simulink model "IFSSIM_TireSuspension"  (R2025b)
settings: Solver=ode1  StartTime=0  StopTime=inf  FixedStep=0.0010416666666666671  RelTol=1e-3
undefined symbols (not defined in the file or in its folder): IFSSIM_aF, IFSSIM_arbF, IFSSIM_arbR, IFSSIM_bR, IFSSIM_camF, IFSSIM_camR, IFSSIM_cgainF, IFSSIM_cgainR, IFSSIM_CoGH, IFSSIM_Crr, IFSSIM_cw, IFSSIM_FzF, IFSSIM_FzR, IFSSIM_Iw, IFSSIM_kwF, IFSSIM_kwR, IFSSIM_L0, IFSSIM_mu, IFSSIM_Ppres, IFSSIM_Rw, IFSSIM_tF, IFSSIM_tR, IFSSIM_Ts, IFSSIM_vreg, IFSSIM_wreg
libraries: vehdynlibtire x1
settings Model: Creator=raulmoran  LastModifiedBy=raulmoran
settings DataIOCC: SignalLoggingName=tsLog

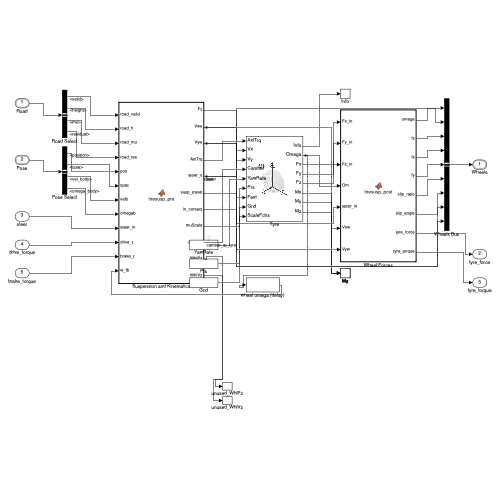
[thumbnail: Simulink's stored preview of the top-level diagram]
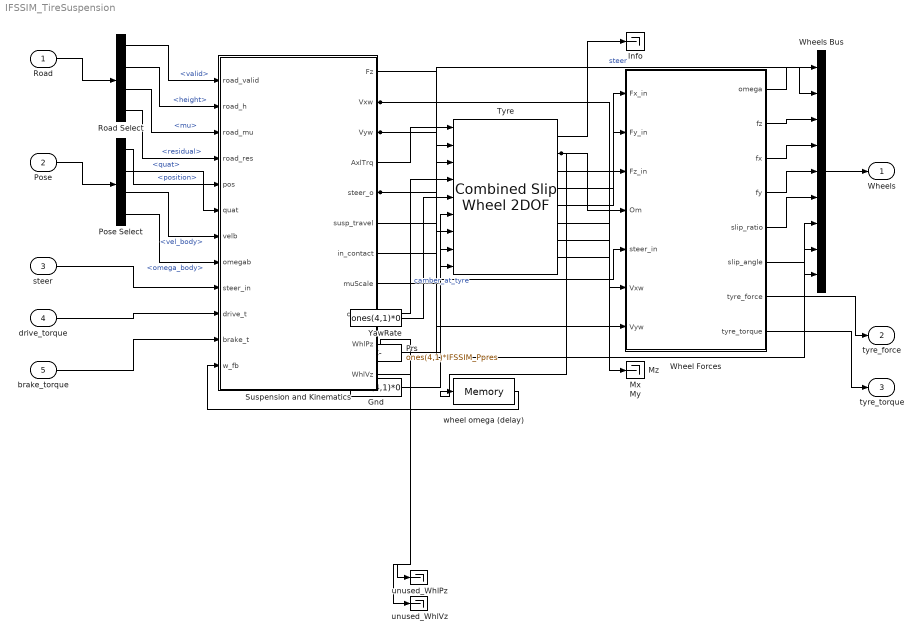
== system IFSSIM_TireSuspension ==
  Road : Inport  OutDataTypeStr=Bus: IFSSIM_RoadBus  BusOutputAsStruct=on
  Pose : Inport  Port=2  OutDataTypeStr=Bus: IFSSIM_PoseBus  BusOutputAsStruct=on
  steer : Inport  Port=3  PortDimensions=4
  drive_torque : Inport  Port=4  PortDimensions=4
  brake_torque : Inport  Port=5  PortDimensions=4
  Gnd : Constant  Value=ones(4,1)*0
  Info : Terminator
  Mx : Terminator
  My : Terminator
  Mz : Terminator
  Pose Select : BusSelector  OutputSignals=position,quat,vel_body,omega_body
  Prs : Constant  Value=ones(4,1)*IFSSIM_Ppres
  Road Select : BusSelector  OutputSignals=valid,height,mu,residual
  Suspension and Kinematics : MATLAB Function  TreatAsAtomicUnit=on
  Tyre : vehdynlibtire/Combined Slip Wheel 2DOF  tireType=External file  tireParamSet=ifssim_tyre.mat  vertType=None  plySteer=off  turnslip=off  BrakeType=None  mu_static=.3  mu_kinetic=.2  drum_abore=0.0508  drum_a=0.123  drum_c=0.212  drum_r=0.15  drum_theta1=0  drum_theta2=126  disk_abore=.05  Rm=.177  num_pads=2  brake_p_bpt=[1 11.4736842105263 21.9473684210526 32.4210526315789 42.8947368421053 53.3684210526316 63.8421052631579 74.3157894736842 84.7894736842105 95.2631578947368 105.736842105263 116.210526315789 126.684210526316 137.157894736842 147.631578947368 158.105263157895 168.578947368421 179.052631578947 189.526315789474 200]  brake_n_bpt=[0 52.6315789473684 105.263157894737 157.894736842105 210.526315789474 263.157894736842 315.789473684211 368.421052631579 421.052631578947 473.684210526316 526.315789473684 578.947368421053 631.578947368421 684.210526315789 736.842105263158 789.473684210526 842.105263157895 894.736842105263 947.368421052632 1000]  f_brake_t=[43.4900602404453 42.5056030554862 41.5350898940194 40.5780454442085 39.6340111501808 38.7025443887544 37.7832176914519 36.8756180088306 35.9793460143796 35.0940154454303 34.2192524787115 33.3546951383474 32.4999927342521 31.6548053290159 30.8188032315107 29.991666515561 29.1730845621415 28.362755623661 27.5603864089927 26.765691687993;498.991217495636 487.695866636631 476.560505099801 465.579679307235 454.748127933653 444.060772460445 433.51270824929 423.099196101319 412.81565427025 402.657650900201 392.620896861006 382.701238955775 372.894653477208 363.197240090814 353.605216024701 344.114910546964 334.722759712992 325.425301366216 316.219170376863 307.10109410434;954.492374750826 932.886130217776 911.585920305583 890.581313170261 869.862244717126 849.419000532136 829.242198807128 809.322774193808 789.651962526121 770.221286354971 751.0225412433 732.047782773203 713.289314220164 694.739674852612 676.391628817892 658.238154578366 640.272434863842 622.48784710877 604.877954344734 587.436496520688;1409.99353200602 1378.07639379892 1346.61133551136 1315.58294703329 1284.9763615006 1254.77722860383 1224.97168936497 1195.5463522863 1166.48827078199 1137.78492180974 1109.42418562559 1081.39432659063 1053.68397496312 1026.28210961441 999.178041611083 972.361398609768 945.822110014692 919.550392851325 893.536738312604 867.771898937035;1865.49468926121 1823.26665738007 1781.63675071715 1740.58458089631 1700.09047828407 1660.13545667552 1620.7011799228 1581.76993037878 1543.32457903786 1505.34855726451 1467.82583000789 1430.74087040806 1394.07863570608 1357.82454437621 1321.96445440427 1286.48464264117 1251.37178516554 1216.61293859388 1182.19552228048 1148.10730135338;2320.9958465164 2268.45692096121 2216.66216592293 2165.58621475934 2115.20459506754 2065.49368474721 2016.43067048064 1967.99350847127 1920.16088729373 1872.91219271928 1826.22747439018 1780.08741422549 1734.47329644903 1689.36697913801 1644.75086719747 1600.60788667257 1556.92146031639 1513.67548433643 1470.85430624835 1428.44270376973;2776.49700377159 2713.64718454235 2651.68758112871 2590.58784862237 2530.31871185102 2470.8519128189 2412.16016103848 2354.21708656376 2296.9971955496 2240.47582817405 2184.62911877248 2129.43395804292 2074.86795719199 2020.9094138998 1967.53727999066 1914.73113070398 1862.47113546724 1810.73803007899 1759.51309021622 1708.77810618608;3231.99816102678 3158.8374481235 3086.71299633449 3015.58948248539 2945.43282863449 2876.21014089059 2807.88965159632 2740.44066465625 2673.83350380547 2608.03946362882 2543.03076315477 2478.78050186034 2415.26261793494 2352.4518486616 2290.32369278385 2228.85437473538 2168.02081061809 2107.80057582154 2048.17187418409 1989.11350860242;3687.49931828197 3604.02771170464 3521.73841154027 3440.59111634842 3360.54694541796 3281.56836896228 3203.61914215416 3126.66424274874 3050.66981206134 2975.60309908359 2901.43240753707 2828.12704567777 2755.6572786779 2683.9942834234 2613.11010557704 2542.97761876678 2473.57048576894 2404.8631215641 2336.83065815196 2269.44891101877;4143.00047553716 4049.21797528579 3956.76382674606 3865.59275021144 3775.66106220143 3686.92659703397 3599.34863271199 3512.88782084123 3427.50612031721 3343.16673453836 3259.83405191936 3177.4735894952 3096.05193942085 3015.5367181852 2935.89651837023 2857.10086279818 2779.12016091979 2701.92566730665 2625.48944211983 2549.78431343512;4598.50163279235 4494.40823886693 4391.78924195184 4290.59438407447 4190.77517898491 4092.28482510566 3995.07812326983 3899.11139893372 3804.34242857308 3710.73036999313 3618.23569630166 3526.82013331263 3436.44660016381 3347.079152947 3258.68293116342 3171.22410682959 3084.66983607064 2998.98821304921 2914.1482260877 2830.11971585147;5054.00279004754 4939.59850244808 4826.81465715762 4715.59601793749 4605.88929576838 4497.64305317735 4390.80761382767 4285.3349770262 4181.17873682896 4078.2940054479 3976.63734068395 3876.16667713006 3776.84126090677 3678.62158770879 3581.46934395661 3485.34735086099 ...(+2764 chars)]  NOMPRES=83000  PRESMAX=166000  PRESMIN=41500  FNOMIN=674.4375  FZMAX=6744.375  FZMIN=0  VXLOW=1  KPUMAX=1.5  KPUMIN=-1.5  ALPMAX=1.570796326794897  ALPMIN=-1.570796326794897  CAMMAX=0.2  CAMMIN=-0.2  LONGVL=1000  FxRelFreqLwrLim=200*pi  FyRelFreqLwrLim=200*pi  MyRelFreqLwrLim=100*pi  omegao=0  UNLOADED_RADIUS=IFSSIM_Rw  WIDTH=0.19  RIM_RADIUS=0.12524  ASPECT_RATIO=0.45  MASS=5  IYY=IFSSIM_Iw  br=0  GRAVITY=-9.81  zo=0  zdoto=0  BREFF=0  DREFF=0  FREFF=0  Q_RE0=1  Q_V1=0  Q_V2=0  Q_FZ1=0  Q_FZ2=0  Q_FZ3=0  Q_FCX=0  Q_FCY=0  Q_FCY2=0  PFZ1=0  VERTICAL_STIFFNESS=1000000000  VERTICAL_DAMPING=0  BOTTOM_OFFST=0  BOTTOM_STIFF=0  Q_CAM1=0  Q_CAM2=0  Q_CAM3=0  Q_FYS1=0  Q_FYS2=0  Q_FYS3=0  LONGITUDINAL_STIFFNESS=96312.41321625  LATERAL_STIFFNESS=44063.25  PCFX1=0  PCFX2=0  PCFX3=0  PCFY1=0  PCFY2=0  PCFY3=0  Q_RA1=0  Q_RA2=0  Q_RB1=0  Q_RB2=0  PCX1=1.46  PDX1=1.4  PDX2=-0.15  PDX3=0  PEX1=-0.5  PEX2=0  PEX3=0  PEX4=0  PKX1=28.560812  PKX2=0  PKX3=0  PHX1=0  PHX2=0  PVX1=0  PVX2=0  PPX1=0  PPX2=0  PPX3=0  PPX4=0  RBX1=9.171685466801819  RBX2=0  RBX3=0  RCX1=1  REX1=0  REX2=0  RHX1=0  QSX1=0  QSX2=0  QSX3=0  QSX4=0  QSX5=0  QSX6=0  QSX7=0  QSX8=0  QSX9=0  QSX10=0  QSX11=0  QSX12=0  QSX13=0  QSX14=0  PPMX1=0  PCY1=1.4  PDY1=1.4  PDY2=-0.15  PDY3=0  PEY1=-0.3  PEY2=0  PEY3=0  PEY4=0  PEY5=0  PKY1=-24.5  PKY2=2  PKY3=0  PKY4=2  PKY5=0  PKY6=0  PKY7=0  PHY1=0  PHY2=0  PVY1=0  PVY2=0  PVY3=0  PVY4=0  PPY1=0  PPY2=0  PPY3=0  PPY4=0  PPY5=0  RBY1=10.84762403199215  RBY2=0  RBY3=0  RBY4=0  RCY1=1  REY1=0  REY2=0  RHY1=0  RHY2=0  RVY1=0  RVY2=0  RVY3=0  RVY4=0  RVY5=0  RVY6=0  QSY1=0  QSY2=0  QSY3=0  QSY4=0  QSY5=0  QSY6=0  QSY7=0  QSY8=0  QBZ1=0  QBZ2=0  QBZ3=0  QBZ4=0  QBZ5=0  QBZ6=0  QBZ9=0  QBZ10=0  QCZ1=0  QDZ1=0  QDZ2=0  QDZ3=0  QDZ4=0  QDZ6=0  QDZ7=0  QDZ8=0  QDZ9=0  QDZ10=0  QDZ11=0  QEZ1=0  QEZ2=0  QEZ3=0  QEZ4=0  QEZ5=0  QHZ1=0  QHZ2=0  QHZ3=0  QHZ4=0  PPZ1=0  PPZ2=0  SSZ1=0  SSZ2=0  SSZ3=0  SSZ4=0  PDXP1=0  PDXP2=0  PDXP3=0  PKYP1=0  PDYP1=0  PDYP2=0  PDYP3=0  PDYP4=0  PHYP1=0  PHYP2=0  PHYP3=0  PHYP4=0  PECP1=0  PECP2=0  QDTP1=0  QCRP1=0  QCRP2=0  QBRP1=0  QDRP1=0  QDRP2=0  aMode=2
  Wheel Forces : MATLAB Function  TreatAsAtomicUnit=on
  Wheels Bus : BusCreator  Inputs=9  OutDataTypeStr=Bus: IFSSIM_WheelsBus  NonVirtualBus=on
  YawRate : Constant  Value=ones(4,1)*0
  unused_WhlPz : Terminator
  unused_WhlVz : Terminator
  wheel omega (delay) : Memory
  Wheels : Outport  OutDataTypeStr=Bus: IFSSIM_WheelsBus
  tyre_force : Outport  Port=2  PortDimensions=3
  tyre_torque : Outport  Port=3  PortDimensions=3
  wires:
  Road/1 -> Road Select/1
  Pose/1 -> Pose Select/1
  Wheels Bus/1 -> Wheels/1
  Road Select/1 -> Suspension and Kinematics/1(road_valid)  "<valid>"
  Road Select/2 -> Suspension and Kinematics/2(road_h)  "<height>"
  Road Select/3 -> Suspension and Kinematics/3(road_mu)  "<mu>"
  Road Select/4 -> Suspension and Kinematics/4(road_res)  "<residual>"
  Pose Select/1 -> Suspension and Kinematics/5(pos)  "<position>"
  Pose Select/2 -> Suspension and Kinematics/6(quat)  "<quat>"
  Pose Select/3 -> Suspension and Kinematics/7(velb)  "<vel_body>"
  Pose Select/4 -> Suspension and Kinematics/8(omegab)  "<omega_body>"
  steer/1 -> Suspension and Kinematics/9(steer_in)
  drive_torque/1 -> Suspension and Kinematics/10(drive_t)
  brake_torque/1 -> Suspension and Kinematics/11(brake_t)
  wheel omega (delay)/1 -> Suspension and Kinematics/12(w_fb)
  Suspension and Kinematics/4(AxlTrq) -> Tyre/1
  Suspension and Kinematics/2(Vxw) -> Tyre/2, Wheel Forces/6(Vxw)
  Suspension and Kinematics/3(Vyw) -> Tyre/3, Wheel Forces/7(Vyw)
  Suspension and Kinematics/9(camber) -> Tyre/4  "camber_at_tyre"
  Suspension and Kinematics/10(WhlPz) -> unused_WhlPz/1
  Suspension and Kinematics/11(WhlVz) -> unused_WhlVz/1
  YawRate/1 -> Tyre/5
  Prs/1 -> Tyre/6
  Suspension and Kinematics/1(Fz) -> Tyre/7
  Gnd/1 -> Tyre/8
  Suspension and Kinematics/8(muScale) -> Tyre/9
  Tyre/1 -> Info/1
  Tyre/2 -> wheel omega (delay)/1, Wheel Forces/4(Om)
  Tyre/3 -> Wheel Forces/1(Fx_in)
  Tyre/4 -> Wheel Forces/2(Fy_in)
  Tyre/5 -> Wheel Forces/3(Fz_in)
  Suspension and Kinematics/5(steer_o) -> Wheel Forces/5(steer_in), Wheels Bus/2  "steer"
  Wheel Forces/1(omega) -> Wheels Bus/1
  Wheel Forces/2(fz) -> Wheels Bus/3
  Wheel Forces/3(fx) -> Wheels Bus/4
  Wheel Forces/4(fy) -> Wheels Bus/5
  Wheel Forces/5(slip_ratio) -> Wheels Bus/6
  Wheel Forces/6(slip_angle) -> Wheels Bus/7
  Suspension and Kinematics/6(susp_travel) -> Wheels Bus/8
  Suspension and Kinematics/7(in_contact) -> Wheels Bus/9
  Wheel Forces/7(tyre_force) -> tyre_force/1
  Wheel Forces/8(tyre_torque) -> tyre_torque/1
  Tyre/6 -> Mx/1
  Tyre/7 -> My/1
  Tyre/8 -> Mz/1

== matlab function IFSSIM_TireSuspension/Wheel Forces ==
  data: Fx_in input size=4; omega output size=4; Fy_in input size=4; Fz_in input size=4; Om input size=4; steer_in input size=4; Vxw input size=4; Vyw input size=4; fz output size=4; fx output size=4; fy output size=4; slip_ratio output size=4; slip_angle output size=4; tyre_force output size=3; tyre_torque output size=3; IFSSIM_aF parameter size=1; IFSSIM_bR parameter size=1; IFSSIM_tF parameter size=1; IFSSIM_tR parameter size=1; IFSSIM_Rw parameter size=1; IFSSIM_vreg parameter size=1; IFSSIM_CoGH parameter size=1
function [omega, fz, fx, fy, slip_ratio, slip_angle, tyre_force, tyre_torque] = ...
         tiresusp_post(Fx_in, Fy_in, Fz_in, Om, steer_in, Vxw, Vyw, IFSSIM_aF, IFSSIM_bR, IFSSIM_tF, IFSSIM_tR, IFSSIM_Rw, IFSSIM_vreg, IFSSIM_CoGH)
%#codegen
% Four wheel forces, in their own wheel frames, assembled into one body-frame
% wrench -- plus the reported per-wheel state.

rx = [ IFSSIM_aF;  IFSSIM_aF; -IFSSIM_bR; -IFSSIM_bR];
ry = [ IFSSIM_tF/2; -IFSSIM_tF/2;  IFSSIM_tR/2; -IFSSIM_tR/2];
Rw = IFSSIM_Rw;

omega = reshape(Om,    4, 1);
fx    = reshape(Fx_in, 4, 1);
fy    = reshape(Fy_in, 4, 1);
fz    = reshape(Fz_in, 4, 1);

slip_ratio = zeros(4,1);  slip_angle = zeros(4,1);
F_sum = zeros(3,1);       M_sum      = zeros(3,1);

for i = 1:4
    % Slip is REPORTED here, not used. The tyre block computes its own
    % internally, with relaxation; this is the algebraic value, recomputed
    % for telemetry so the bus still carries the quantity it always did.
    vref = max(abs(Vxw(i)), IFSSIM_vreg);
    slip_ratio(i) = (omega(i)*Rw - Vxw(i)) / vref;
    slip_angle(i) = atan2(Vyw(i), vref);

    % Wheel frame -> body frame. Fx acts along the wheel, Fy across it, and
    % the wheel is rotated by the steer angle relative to the body.
    d  = steer_in(i);
    cd = cos(d); sd = sin(d);
    Fb = [fx(i)*cd - fy(i)*sd; fx(i)*sd + fy(i)*cd; fz(i)];
    F_sum = F_sum + Fb;

    % The tyre force acts at the CONTACT PATCH, on the road, not at the CoG.
    % That arm IS load transfer: it is what turns a lateral force into a roll
    % moment and a longitudinal force into a pitch moment.
    %
    % This used to be [rx; ry; 0], and the reason it survived so long is that
    % a zero z still gives the RIGHT answer for three of the six terms. Yaw
    % (rx*fy - ry*fx) has no z in it at all, and the roll and pitch from the
    % VERTICAL loads (ry*fz, -rx*fz) do not either. So the car rolled
    % correctly whenever something else rolled it -- which is every test that
    % imposes a body rate. What it could not do was roll ITSELF: the two
    % missing terms, -rz*fy and +rz*fx, are precisely the ones by which the
    % tyres act on the body. Measured before the fix: 0.000000 rad of roll in
    % a 1.2 g corner, and load transfer at 0.1% of what m*a*h/t requires.
    %
    % Taking the arm all the way to the ground puts the roll centre at ground
    % level, so every newton of lateral transfer goes through the springs and
    % none through the suspension links. That is a real assumption and it is
    % stated here rather than hidden: this model HAS no links -- no wishbones,
    % no instantaneous centres -- so a non-zero roll centre would not be a
    % better number, it would be an invented one. It costs less than it
    % sounds: the TOTAL transfer is m*a*h/t whatever the roll centre does.
    % What a real one would change is the elastic/geometric split, and with
    % it the roll ANGLE and the transient, not the steady-state load split.
    %
    % The height is held constant at the static CoG height. Tracking ride
    % height through suspension travel would be a centimetre of correction on
    % a 34 cm arm, sitting on top of a CoG height nobody has measured.
    M_sum = M_sum + cross([rx(i); ry(i); -IFSSIM_CoGH], Fb);
end

tyre_force  = F_sum;
tyre_torque = M_sum;
end

== matlab function IFSSIM_TireSuspension/Suspension and Kinematics ==
  data: road_valid input size=4; Fz output size=4; road_h input size=4; road_mu input size=4; road_res input size=4; pos input size=3; quat input size=4; velb input size=3; omegab input size=3; steer_in input size=4; drive_t input size=4; brake_t input size=4; w_fb input size=4; Vxw output size=4; Vyw output size=4; AxlTrq output size=4; steer_o output size=4; susp_travel output size=4; in_contact output size=4; muScale output size=[27 4]; camber output size=4; WhlPz output size=4; WhlVz output size=4; IFSSIM_arbF parameter size=1; IFSSIM_arbR parameter size=1; IFSSIM_Ts parameter size=1; IFSSIM_Iw parameter size=1; IFSSIM_wreg parameter size=1; IFSSIM_aF parameter size=1; IFSSIM_bR parameter size=1; IFSSIM_tF parameter size=1; IFSSIM_tR parameter size=1; IFSSIM_Rw parameter size=1; IFSSIM_kwF parameter size=1; IFSSIM_kwR parameter size=1; IFSSIM_cw parameter size=1; IFSSIM_L0 parameter size=1; IFSSIM_FzF parameter size=1; IFSSIM_FzR parameter size=1; IFSSIM_camF parameter size=1; IFSSIM_camR parameter size=1; IFSSIM_cgainF parameter size=1; IFSSIM_cgainR parameter size=1; IFSSIM_mu parameter size=1; IFSSIM_Crr parameter size=1
function [Fz, Vxw, Vyw, AxlTrq, steer_o, susp_travel, in_contact, muScale, camber, WhlPz, WhlVz] = ...
         tiresusp_pre(road_valid, road_h, road_mu, road_res, pos, quat, velb, omegab, steer_in, drive_t, brake_t, w_fb, IFSSIM_arbF, IFSSIM_arbR, IFSSIM_Ts, IFSSIM_Iw, IFSSIM_wreg, IFSSIM_aF, IFSSIM_bR, IFSSIM_tF, IFSSIM_tR, IFSSIM_Rw, IFSSIM_kwF, IFSSIM_kwR, IFSSIM_cw, IFSSIM_L0, IFSSIM_FzF, IFSSIM_FzR, IFSSIM_camF, IFSSIM_camR, IFSSIM_cgainF, IFSSIM_cgainR, IFSSIM_mu, IFSSIM_Crr)
%#codegen
% Suspension load and contact-patch kinematics for four corners, plus the
% axle torque that drives the tyre block.
%
% Wheel order FL, FR, RL, RR. Body frame ISO 8855: x forward, y LEFT, z up.

Rw = IFSSIM_Rw;

% Wheel positions in the body frame, at CoG height. y is POSITIVE LEFT, so the
% left wheels take +track/2. Getting this backwards mirrors the car and is
% almost impossible to see in a lap time.
rx = [ IFSSIM_aF;  IFSSIM_aF; -IFSSIM_bR; -IFSSIM_bR];
ry = [ IFSSIM_tF/2; -IFSSIM_tF/2;  IFSSIM_tR/2; -IFSSIM_tR/2];
Fz_static = [IFSSIM_FzF; IFSSIM_FzF; IFSSIM_FzR; IFSSIM_FzR];

q = quat / max(norm(quat), eps);
R = q2r(q);                      % body -> world
vel_world   = R * velb;
omega_world = R * omegab;

Fz      = zeros(4,1);  Vxw     = zeros(4,1);  Vyw        = zeros(4,1);
AxlTrq  = zeros(4,1);  steer_o = zeros(4,1);  susp_travel= zeros(4,1);
camber  = zeros(4,1);
% What the VDB suspension block wants, if it is in the model: displacement
% from the static ride position in a z-DOWN frame, so positive is droop and
% our compression-positive delta is its negative. Measured, see
% docs/vdb_step1_port_semantics.md -- feeding it a ride height instead of a
% displacement is what made the first attempt return 2568 N a wheel.
WhlPz   = zeros(4,1);  WhlVz = zeros(4,1);
in_contact = zeros(4,1);  muScale = ones(27,4);

% ---- suspension deflection, all four corners at once ----------------
% This has to be a separate pass. An anti-roll bar reacts the DIFFERENCE in
% deflection across an axle, so no corner's vertical load can be known until
% both corners of its axle are.
delta  = zeros(4,1);
ddelta = zeros(4,1);
for i = 1:4
    r_w = R * [rx(i); ry(i); 0];
    p_w = pos + r_w;                      % corner position, world
    % delta > 0 means compressed relative to static ride height.
    gap       = p_w(3) - (road_h(i) + Rw);    % attachment above wheel centre
    delta(i)  = IFSSIM_L0 - gap;
    % Compression RATE is the downward velocity of this corner. Using the
    % corner velocity rather than the CoG velocity is what makes roll and
    % pitch damping appear at all.
    v_corner  = vel_world + cross(omega_world, r_w);
    ddelta(i) = -v_corner(3);
end

% ---- anti-roll bars -------------------------------------------------
% A bar carries K_arb times the roll angle of its axle, delivered as a force
% couple across the track: dF = K_arb*(dL - dR)/t^2, up on the compressed
% side and down on the other, summing to zero so it adds no heave stiffness.
%
% These are not a detail. They are the ONLY thing that makes the front and
% rear roll stiffnesses differ, and that difference is the car's balance.
% With four equal springs and equal tracks -- which is what this model had --
% lateral load transfer splits exactly 50.0/50.0 at every steer angle and
% nothing can move it, so the car can be neither understeering nor
% oversteering by construction. See ifssim_params for how the bar rates come
% out of RollStiffnessFront/Rear, which until now were read by nothing.
arbF = IFSSIM_arbF * (delta(1) - delta(2)) / (IFSSIM_tF*IFSSIM_tF);
arbR = IFSSIM_arbR * (delta(3) - delta(4)) / (IFSSIM_tR*IFSSIM_tR);
arb  = [arbF; -arbF; arbR; -arbR];

% ---- camber -----------------------------------------------------------
% Inclination each tyre sees: its static setting, plus the share of body roll
% the geometry does NOT take back out. Camber gain 1.0 keeps the wheel
% upright through the corner; a real double wishbone falls short of that.
%
% Roll comes from the quaternion the chassis already integrates, so this is
% the roll the car ACTUALLY has -- not the algebraic estimate the design
% model has to make. That is the one place the plant is now ahead of it.
%
% It is wired to the tyre block's Camber input, which this model used to hold
% at a constant zero. The tyre does not yet RESPOND to it: the camber
% coefficients in the Magic Formula set are zeroed, because nobody has put
% this tyre on a rig and inventing PDY3 would be inventing grip. The
% kinematics are real and arrive at the tyre; the tyre's answer to them is
% the part still waiting on data.
%
% The two terms mirror DIFFERENTLY, and getting that backwards is the easy
% mistake. In the ISO tyre axis system y points left on BOTH wheels, so:
%
%   static camber is symmetric in space -- the tops lean toward each other --
%   and therefore reads with OPPOSITE sign on the two sides (sgnOut);
%
%   roll tilts both wheels the SAME way in space, so it reads with the SAME
%   sign on both, and must stay OUTSIDE the mirror.
%
% This used to apply the static setting uniformly to all four and mirror the
% roll term -- exactly inverted, on both counts. It changed no force, because
% the camber coefficients are zeroed, and it would have changed every one of
% them the day rig data arrives. The structure here is not argued from the
% convention: it is what the VDB double-wishbone block measurably does
% (see vdb_camber_mask), and the two now agree to 3e-10 deg.
%
% The OVERALL SIGN of gamma is still unpinned. Nothing in this plant can
% settle it while the Magic Formula camber terms are zero -- there is no
% observable to check it against. It wants fixing against rig data, not
% against an argument.
rollAng = atan2(2*(q(1)*q(2) + q(3)*q(4)), 1 - 2*(q(2)*q(2) + q(3)*q(3)));
sgnOut  = [-1; 1; -1; 1];
camber  = sgnOut .* [IFSSIM_camF; IFSSIM_camF; IFSSIM_camR; IFSSIM_camR] + ...
          (1 - [IFSSIM_cgainF; IFSSIM_cgainF; IFSSIM_cgainR; IFSSIM_cgainR]) * rollAng;

for i = 1:4
    r_b = [rx(i); ry(i); 0];
    r_w = R * r_b;
    p_w = pos + r_w;                      % corner position, world

    kw_i = IFSSIM_kwF; if i > 2, kw_i = IFSSIM_kwR; end
    Fz_i = Fz_static(i) + kw_i * delta(i) + IFSSIM_cw * ddelta(i) + arb(i);

    % A tyre cannot pull the road. Clamping here is what lets a wheel lift
    % in a corner instead of generating negative grip.
    if Fz_i < 0, Fz_i = 0; end
    % Contact needs the platform to have actually CHARACTERISED the ground,
    % not merely to have hit something with one ray.
    %
    % A NEGATIVE residual is the platform saying it could not fit a plane at
    % all - fewer than three of its rays hit - so it does not know what is
    % under this wheel. Standing on an answer nobody has is how a wheel ends
    % up loaded against geometry that is not there.
    %
    % A LARGE residual is a different thing entirely and deliberately does NOT
    % remove contact. It means the patch spans a step or a kerb edge: the
    % ground is poorly described by a plane, but the tyre is still touching
    % it. Dropping Fz there would make the car fall through every kerb, which
    % is worse than the flat-plane approximation it would be replacing.
    fit_known = (road_res(i) >= 0);
    contact = (road_valid(i) > 0.5) && (Fz_i > 0) && fit_known;
    if ~contact, Fz_i = 0; end

    % ---- contact-patch velocity ------------------------------------
    v_b = velb + cross(omegab, r_b);
    d   = steer_in(i);
    cd  = cos(d); sd = sin(d);
    vx =  v_b(1)*cd + v_b(2)*sd;          % along the wheel
    vy = -v_b(1)*sd + v_b(2)*cd;          % across it

    % ---- axle torque -----------------------------------------------
    % The tyre block's own brake and rolling-resistance models are switched
    % off, so both arrive here as torque on the axle instead.
    %
    % w_fb is last step's wheel speed, delayed. Using it rather than the
    % block's live Omega is what keeps this out of an algebraic loop; at
    % 1/960 s the wheel cannot turn far enough in one step for the
    % difference to matter.
    %
    % tanh, not sign: sign() chatters about zero every step at 1/960 s. tanh
    % also means both torques fade smoothly to zero as the wheel stops, so
    % they RESIST motion but cannot HOLD a stopped car - arresting creep
    % entirely needs a stiction term, which this is not.
    % Smoothed over IFSSIM_wreg, which is deliberately WIDER than the wheel
    % speed one step of brake torque can produce. Narrower than that and this
    % is sign() in all but name, and the stop ends in a limit cycle.
    dirw    = tanh(w_fb(i) / IFSSIM_wreg);
    % LOCK, DO NOT REVERSE. Brake torque is a magnitude opposing rotation, so
    % it must never be large enough to drive the wheel backwards through zero.
    % The old hand-written tyre clamped the wheel state directly after
    % integrating; wheel spin now lives inside the tyre block, where we cannot
    % reach it, so the limit has to be applied to the TORQUE instead.
    %
    % Iw*|w|/Ts is exactly the torque that brings this wheel to rest in one
    % step. Anything beyond it would reverse the wheel, which a brake cannot
    % do: at 286 N.m on Iw = 0.21 one step moves the wheel 1.4 rad/s, so
    % without this the EBS walks a stopping wheel backwards through zero.
    T_cap   = IFSSIM_Iw * abs(w_fb(i)) / IFSSIM_Ts;
    T_brake = min(brake_t(i), T_cap) * dirw;
    % Rolling resistance. Physically the contact patch's pressure
    % distribution shifts forward of the axle and the resulting moment
    % opposes rotation. Modelling it as a drag force on the chassis would
    % give a similar top speed and the wrong wheel dynamics.
    T_roll  = IFSSIM_Crr * Fz_i * Rw * dirw;
    AxlTrq(i) = drive_t(i) - T_brake - T_roll;

    % ---- friction scaling ------------------------------------------
    % The tyre carries one set of coefficients, but the road can differ under
    % each wheel. Magic Formula takes a column of 27 SCALING FACTORS per
    % wheel, and two of them scale peak friction; everything else stays 1.
    %
    % Indices 3 and 10 are LMUX and LMUY in the standard Magic Formula
    % ordering. That ordering is not documented on the block and the code
    % behind it is P-coded, so it was checked instead of assumed: perturbing
    % each of the 27 in turn, 19 and 20 moved the combined-slip coupling,
    % which is exactly where the standard order puts LXAL and LYKA, and 3
    % scaled lateral grip directly in a pure-slip test. Both mu factors are
    % set to the same ratio, so a road reporting the nominal mu scales by 1.
    muw = road_mu(i);
    if muw <= 0, muw = IFSSIM_mu; end
    mur = muw / IFSSIM_mu;
    muScale(3,i)  = mur;
    muScale(10,i) = mur;

    Fz(i)=Fz_i; Vxw(i)=vx; Vyw(i)=vy; steer_o(i)=d;
    susp_travel(i)=delta(i); in_contact(i)=double(contact);
    WhlPz(i) = -delta(i);  WhlVz(i) = -ddelta(i);
end
end

function R = q2r(q)
%#codegen
w=q(1); x=q(2); y=q(3); z=q(4);
R = [1-2*(y*y+z*z),   2*(x*y-z*w),   2*(x*z+y*w); ...
       2*(x*y+z*w), 1-2*(x*x+z*z),   2*(y*z-x*w); ...
       2*(x*z-y*w),   2*(y*z+x*w), 1-2*(x*x+y*y)];
end
